simulink model "PI_stability_test"  (R2017a)
settings: Solver=VariableStepAuto  StartTime=0.0  StopTime=0.8  RelTol=1e-3
settings Model: Creator=Dell  LastModifiedBy=Dell

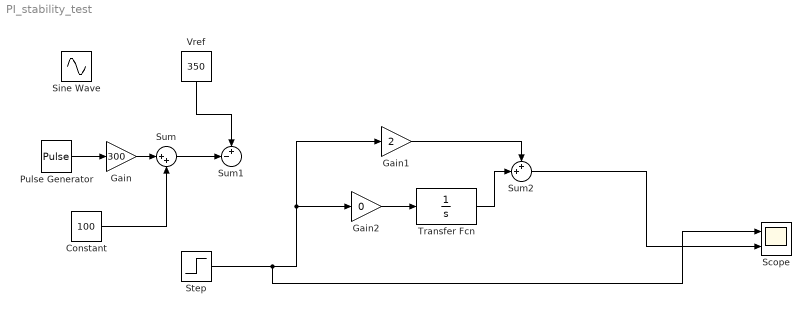
== system PI_stability_test ==
  Constant : Constant  Value=100
  Gain : Gain  Gain=300
  Gain1 : Gain  Gain=2
  Gain2 : Gain  Gain=0
  Pulse Generator : DiscretePulseGenerator  PulseType=Time based  Period=.2  PulseWidth=50
  Scope : Scope  NumInputPorts=2
  Sine Wave : Sin  Frequency=2*pi*1000  SampleTime=0
  Step : Step  Time=0.1  SampleTime=0
  Sum : Sum  Inputs=|++
  Sum1 : Sum  Inputs=+-|
  Sum2 : Sum  Inputs=++|
  Transfer Fcn : TransferFcn  Denominator=[1 0]
  Vref : Constant  Value=350
  wires:
  Vref/1 -> Sum1/1
  Sum2/1 -> Scope/2
  Sum/1 -> Sum1/2
  Constant/1 -> Sum/2
  Gain/1 -> Sum/1
  Pulse Generator/1 -> Gain/1
  Gain2/1 -> Transfer Fcn/1
  Gain1/1 -> Sum2/1
  Transfer Fcn/1 -> Sum2/2
  Step/1 -> Scope/1, Gain2/1, Gain1/1
